simulink library "inductance"  (R2024a)
settings: Solver=VariableStepAuto  StartTime=0.0  StopTime=10.0  RelTol=1e-3
settings Model: Creator=Bocchio  LastModifiedBy=Bocchio

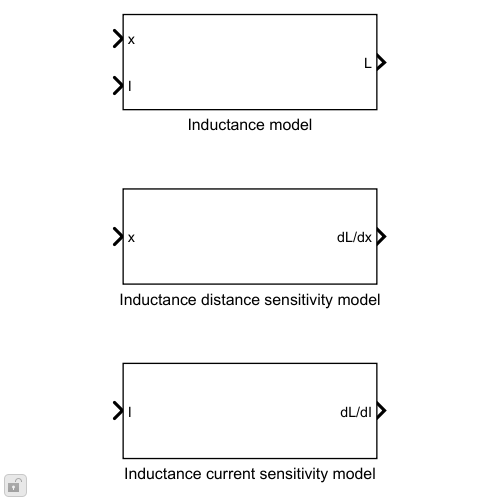
[thumbnail: Simulink's stored preview of the top-level diagram]
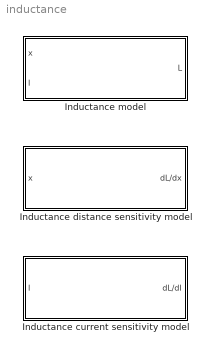
== system inductance ==
  Inductance current sensitivity model : Subsystem  mask{aI=0, bI=0, LI=0}
      mask DialogControl DescGroupVar Prompt: Inductance sensitivity to object current
      mask DialogControl DescTextVar Prompt: Insert the parameters of the inductor
  Inductance distance sensitivity model : Subsystem  mask{ax=0, Lx=0}
      mask DialogControl DescGroupVar Prompt: Inductance sensitivity to object distance
      mask DialogControl DescTextVar Prompt: Insert the parameters of the inductor
  Inductance model : Subsystem  mask(Inductance model){L0=0, ax=0, Lx=0, aI=0, bI=0, LI=0}
      mask DialogControl DescGroupVar Prompt: Inductance model
      mask DialogControl DescTextVar Prompt: Insert the parameters of the inductance

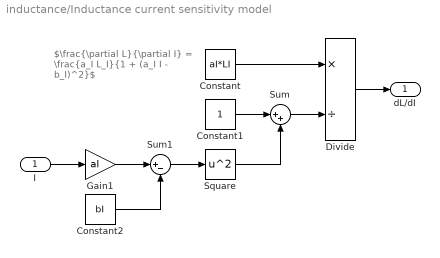
== system inductance/Inductance current sensitivity model ==
  note: $\frac{\partial L}{\partial I} = \frac{a_I L_I}{1 + (a_I I - b_I)^2}$
  I : Inport
  Constant : Constant  Value=aI*LI
  Constant1 : Constant
  Constant2 : Constant  Value=bI
  Divide : Product  Inputs=*/
  Gain1 : Gain  Gain=aI
  Square : Math  Operator=square
  Sum : Sum  Inputs=|++
  Sum1 : Sum  Inputs=|+-
  dL/dI : Outport
  wires:
  Divide/1 -> dL/dI/1
  Constant/1 -> Divide/1
  Square/1 -> Sum/2
  Constant1/1 -> Sum/1
  Sum/1 -> Divide/2
  I/1 -> Gain1/1
  Gain1/1 -> Sum1/1
  Sum1/1 -> Square/1
  Constant2/1 -> Sum1/2

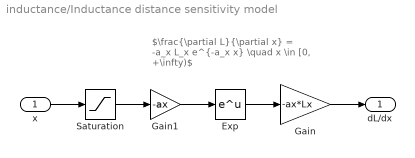
== system inductance/Inductance distance sensitivity model ==
  note: $\frac{\partial L}{\partial x} = -a_x L_x e^{-a_x x} \quad x \in [0, +\infty)$
  x : Inport
  Exp : Math
  Gain : Gain  Gain=-ax*Lx
  Gain1 : Gain  Gain=-ax
  Saturation : Saturate  UpperLimit=+inf  LowerLimit=0
  dL/dx : Outport
  wires:
  Gain1/1 -> Exp/1
  Exp/1 -> Gain/1
  x/1 -> Saturation/1
  Gain/1 -> dL/dx/1
  Saturation/1 -> Gain1/1

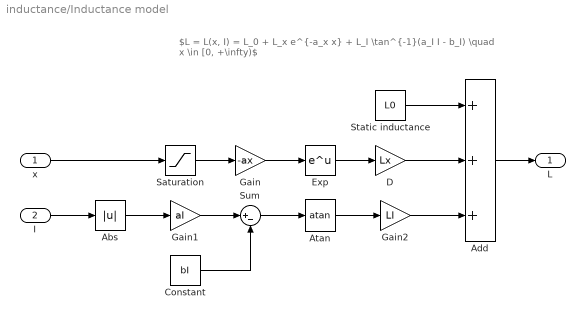
== system inductance/Inductance model ==
  note: $L = L(x, I) = L_0 + L_x e^{-a_x x} + L_I \tan^{-1}(a_I I - b_I) \quad x \in [0, +\infty)$
  x : Inport
  I : Inport  Port=2
  Abs : Abs  SaturateOnIntegerOverflow=off
  Add : Sum  Inputs=+++
  Atan : Trigonometry  Operator=atan  OutputSignalType=real
  Constant : Constant  Value=bI
  D : Gain  Gain=Lx
  Exp : Math
  Gain : Gain  Gain=-ax
  Gain1 : Gain  Gain=aI
  Gain2 : Gain  Gain=LI
  Saturation : Saturate  UpperLimit=+inf  LowerLimit=0
  Static inductance : Constant  Value=L0
  Sum : Sum  Inputs=|+-
  L : Outport
  wires:
  D/1 -> Add/2
  Static inductance/1 -> Add/1
  Exp/1 -> D/1
  Gain/1 -> Exp/1
  x/1 -> Saturation/1
  Saturation/1 -> Gain/1
  Add/1 -> L/1
  I/1 -> Abs/1
  Sum/1 -> Atan/1
  Abs/1 -> Gain1/1
  Gain1/1 -> Sum/1
  Constant/1 -> Sum/2
  Atan/1 -> Gain2/1
  Gain2/1 -> Add/3
